simulink model "Hunt_crossley_MCMC"  (Simulink 8.9)
settings: Solver=ode3  StartTime=0.0  StopTime=25  FixedStep=0.001  RelTol=1e-3  EnableMultiTasking=on
undefined symbols (not defined in the file): sigbuilder_block
libraries: simulink x3, dspstat3 x1
settings Model: Creator=x  LastModifiedBy=x
settings DataIOCC: SignalLoggingSaveFormat=Dataset
settings OptimizationCC: ExpressionDepthLimit=2147483647
settings DebuggingCC: SolverPrmCheckMsg=warning  FcnCallInpInsideContextMsg=error
settings GRTTargetCC: CombineOutputUpdateFcns=on  GRTInterface=off

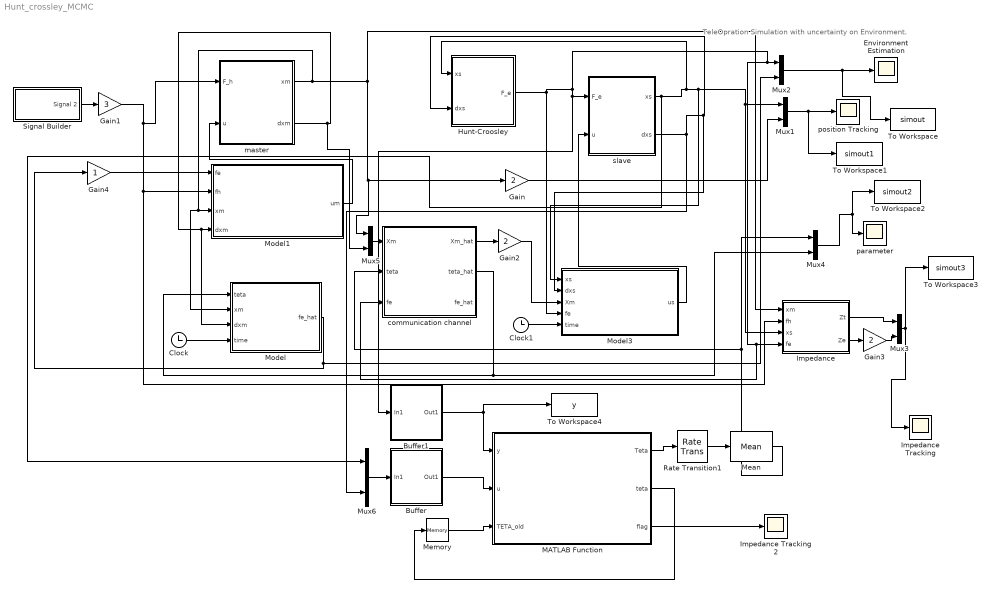
== system Hunt_crossley_MCMC ==
  note: TeleOpration Simulation with uncertainty on Environment.
  Buffer : Subsystem
  Buffer1 : Subsystem
  Clock : Clock
  Clock1 : Clock
  Environment Estimation : Scope
  Gain : Gain  Gain=2
  Gain1 : Gain  Gain=3
  Gain2 : Gain  Gain=2
  Gain3 : Gain  Gain=2
  Gain4 : Gain
  Hunt-Croosley : Subsystem
  Impedance : MATLAB Function  TreatAsAtomicUnit=on
  "Impedance Tracking " : Scope
  Impedance Tracking 2 : Scope
  MATLAB Function : MATLAB Function  TreatAsAtomicUnit=on
  Mean : dspstat3/Mean  run=off  reset_popup=None  InputProcessing=Columns as channels (frame based)  directionMode=Each row  dimension=1  roiEnable=off  roiType=Rectangles  roiPortion=Entire ROI  roiOutput=Individual statistics for each ROI  roiFlag=off  outputDataTypeStr=Inherit: Same as accumulator  outputLastDataTypeStr=Inherit: Same as accumulator  outputMin=[]  outputMax=[]  roundingMode=Floor  overflowMode=off
  Memory : Memory  X0=[1;1 ;1]*ones(1,2000)  InheritSampleTime=on
  Model : MATLAB Function  TreatAsAtomicUnit=on
  Model1 : MATLAB Function  TreatAsAtomicUnit=on
  Model3 : MATLAB Function  TreatAsAtomicUnit=on
  Mux{1..6} (6 alike) : Mux  Inputs=2
  Rate Transition1 : RateTransition  OutPortSampleTime=0.001
  Signal Builder : Subsystem  Tag=STV Subsys  LoadFcn=sigbuilder_block('load');  StartFcn=sigbuilder_block('start');  StopFcn=sigbuilder_block('stop');  ClipboardFcn=sigbuilder_block('clipboard');  mask(Sigbuilder block){tuvar=[0:10]}
      mask help: Simulink:masks:SigbuilderBlock_MD
      mask init:
      | if ~strcmp(get_param(bdroot(gcbh),'SimulationStatus'),'stopped') tuvar = sigbuilder_block('maskInit'); end
      settings: CopyFcn=sigbuilder_block('copy');  DeleteFcn=sigbuilder_block('delete');  ModelCloseFcn=sigbuilder_block('modelClose');  PreSaveFcn=sigbuilder_block('preSave');  PauseFcn=sigbuilder_block('pause');  ContinueFcn=sigbuilder_block('continue');  NameChangeFcn=sigbuilder_block('namechange');  OpenFcn=sigbuilder_block('open',[216 34.1379 544.345 383.586 ]);  CloseFcn=sigbuilder_block('close');
      mask Display: plot(0, 0, 100, 100,[2, 2, 32, 32, 2], [68, 8, 8, 68, 68],[32, 2], [38, 38], [32, 19, 2],[53, 60, 44], [32, 17, 17, 2],[16, 16, 31, 31]);txt = getActiveGroup(gcbh);text(2, 100, txt,'verticalAlignment', 'top');
  To Workspace : ToWorkspace  VariableName=simout  SampleTime=-1
  To Workspace1 : ToWorkspace  VariableName=simout1  SampleTime=-1
  To Workspace2 : ToWorkspace  VariableName=simout2  SampleTime=-1
  To Workspace3 : ToWorkspace  VariableName=simout3  SampleTime=-1
  To Workspace4 : ToWorkspace  VariableName=y  SampleTime=-1
  communication channel : Subsystem
  master : Subsystem
  parameter : Scope
  position Tracking : Scope
  slave : Subsystem
  wires:
  master/1(xm) -> Model/2(xm), Model1/3(xm), Mux5/1, Gain/1, Impedance/1(xm)
  Gain/1 -> Mux1/2
  Mux1/1 -> To Workspace1/1, position Tracking/1
  Impedance/1(Zt) -> Mux3/1
  Mux3/1 -> To Workspace3/1, "Impedance Tracking "/1
  communication channel/1(Xm_hat) -> Gain2/1
  Impedance/2(Ze) -> Gain3/1
  Signal Builder/1(Signal 2) -> Gain1/1
  Gain3/1 -> Mux3/2
  Model1/1(um) -> master/2(u)
  Model3/1(us) -> slave/2(u)
  master/2(dxm) -> Mux5/2, Model/3(dxm), Model1/4(dxm)
  Gain2/1 -> Model3/3(Xm)
  Clock/1 -> Model/4(time)
  communication channel/2(teta_hat) -> Mux4/2, Model/1(teta)
  Mean/1 -> Mux4/1, communication channel/2(teta)
  Mux5/1 -> communication channel/1(Xm)
  Clock1/1 -> Model3/5(time)
  Mux2/1 -> To Workspace/1, Environment Estimation/1
  Mux4/1 -> To Workspace2/1, parameter/1
  Gain1/1 -> master/1(F_h), Model1/2(fh), Impedance/2(fh)
  Model/1(fe_hat) -> Gain4/1, Mux2/2
  Gain4/1 -> Model1/1(fe)
  Mux6/1 -> Buffer/1(In1)
  MATLAB Function/2(teta) -> Memory/1
  Buffer/1(Out1) -> MATLAB Function/2(u)
  Buffer1/1(Out1) -> MATLAB Function/1(y), To Workspace4/1
  Rate Transition1/1 -> Mean/1
  Memory/1 -> MATLAB Function/3(TETA_old)
  MATLAB Function/1(Teta) -> Rate Transition1/1
  Hunt-Croosley/1(F_e) -> Buffer1/1(In1), slave/1(F_e), communication channel/3(fe), Impedance/4(fe), Mux2/1, Model3/4(fe)
  slave/1(xs) -> Mux6/1, Model3/1(xs), Impedance/3(xs), Mux1/1, Hunt-Croosley/1(xs)
  slave/2(dxs) -> Mux6/2, Model3/2(dxs), Hunt-Croosley/2(dxs)
  MATLAB Function/3(flag) -> Impedance Tracking 2/1

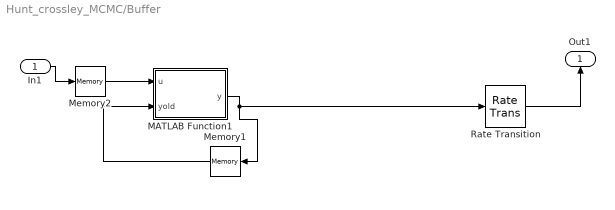
== system Hunt_crossley_MCMC/Buffer ==
  In1 : Inport
  MATLAB Function1 : MATLAB Function  TreatAsAtomicUnit=on
  Memory1 : Memory  X0=zeros(100,2)  LinearizeMemory=on
  Memory2 : Memory  X0=[0;0]  InheritSampleTime=on
  Rate Transition : RateTransition  X0=zeros(100,2)  OutPortSampleTime=0.1
  Out1 : Outport
  wires:
  Rate Transition/1 -> Out1/1
  Memory1/1 -> MATLAB Function1/2(yold)
  In1/1 -> Memory2/1
  MATLAB Function1/1(y) -> Memory1/1, Rate Transition/1
  Memory2/1 -> MATLAB Function1/1(u)

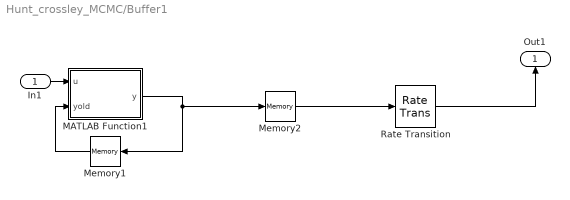
== system Hunt_crossley_MCMC/Buffer1 ==
  In1 : Inport
  MATLAB Function1 : MATLAB Function  TreatAsAtomicUnit=on
  Memory1 : Memory  X0=zeros(100,1)  LinearizeMemory=on
  Memory2 : Memory  X0=zeros(100,1)  LinearizeMemory=on
  Rate Transition : RateTransition  X0=zeros(100,1)  OutPortSampleTime=0.1
  Out1 : Outport
  wires:
  Memory1/1 -> MATLAB Function1/2(yold)
  In1/1 -> MATLAB Function1/1(u)
  Rate Transition/1 -> Out1/1
  MATLAB Function1/1(y) -> Memory2/1, Memory1/1
  Memory2/1 -> Rate Transition/1

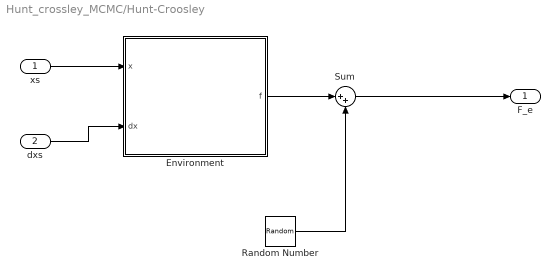
== system Hunt_crossley_MCMC/Hunt-Croosley ==
  xs : Inport
  dxs : Inport  Port=2
  Environment : MATLAB Function  TreatAsAtomicUnit=on
  Random Number : RandomNumber  Variance=0.1
  Sum : Sum  Inputs=|++
  F_e : Outport
  wires:
  xs/1 -> Environment/1(x)
  dxs/1 -> Environment/2(dx)
  Environment/1(f) -> Sum/1
  Sum/1 -> F_e/1
  Random Number/1 -> Sum/2

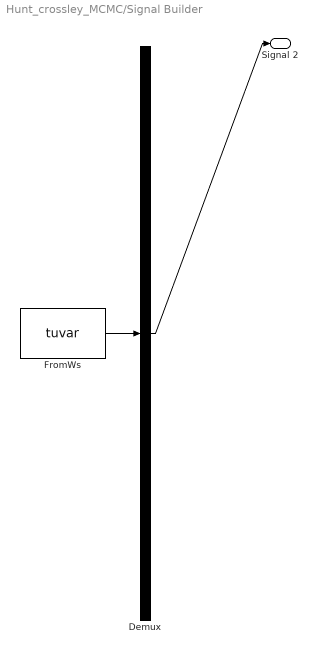
== system Hunt_crossley_MCMC/Signal Builder ==
  Demux : Demux  Tag=STV Demux  Outputs=1
  FromWs : FromWorkspace  Tag=STV FromWs  VariableName=tuvar  SampleTime=0  SigBuilderData=DataTag1  VnvData=DataTag2
      SigBuilderData=|
      | common.afterFinalStr = 'Extrapolate'
      | common.sampleTime = 0
      | dataSet.timeRange = [0 25]
      | dataSet.name = 'Group 1'
      | sbobj.Groups.Name = 'Group 1'
      | sbobj.Groups.Signals.Name = 'Signal 2'
      | sbobj.Groups.Signals.XData = [0 5.05 5.05 15.05 15.05 16.35 16.35 21.05 21.05 25]
      | sbobj.Groups.Signals.YData = [0.49 0.49 1.98 1.98 -0.82 -0.82 0.98 0.98 -0.24 -0.24]
      | sbobj.Groups.TimeRange = [0 25]
  Signal 2 : Outport  Tag=STV Outport
  wires:
  FromWs/1 -> Demux/1
  Demux/1 -> Signal 2/1

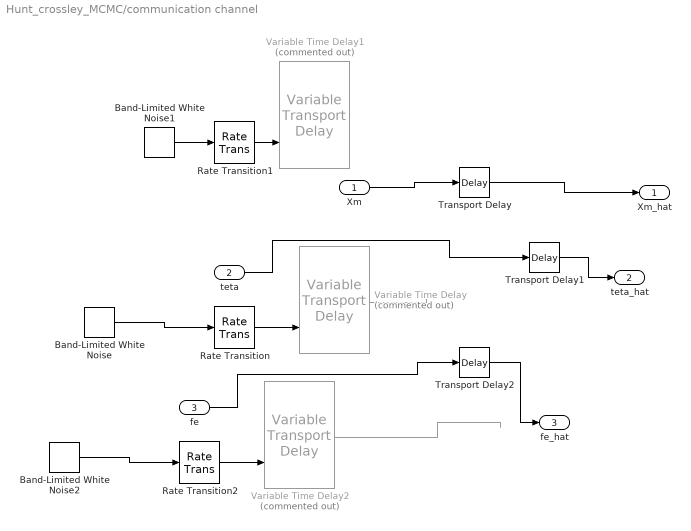
== system Hunt_crossley_MCMC/communication channel ==
  Xm : Inport
  teta : Inport  Port=2
  fe : Inport  Port=3
  Band-Limited White Noise : simulink/Sources/Band-Limited White Noise  Cov=[0.1]  Ts=0.2  seed=[23341]
  Band-Limited White Noise1 : simulink/Sources/Band-Limited White Noise  Cov=[0.1]  Ts=0.2  seed=[5368541]
  Band-Limited White Noise2 : simulink/Sources/Band-Limited White Noise  Cov=[0.1]  Ts=0.2  seed=[28931]
  Rate Transition : RateTransition
  Rate Transition1 : RateTransition
  Rate Transition2 : RateTransition
  Transport Delay : TransportDelay
  Transport Delay1 : TransportDelay
  Transport Delay2 : TransportDelay
  Variable Time Delay : VariableTransportDelay  Commented=on  MaximumDelay=4  TransDelayFeedthrough=on
  Variable Time Delay1 : VariableTransportDelay  Commented=on  MaximumDelay=4  TransDelayFeedthrough=on
  Variable Time Delay2 : VariableTransportDelay  Commented=on  MaximumDelay=4  TransDelayFeedthrough=on
  Xm_hat : Outport
  teta_hat : Outport  Port=2
  fe_hat : Outport  Port=3
  wires:
  Band-Limited White Noise/1 -> Rate Transition/1
  Rate Transition/1 -> Variable Time Delay/2
  Band-Limited White Noise1/1 -> Rate Transition1/1
  Rate Transition1/1 -> Variable Time Delay1/2
  Variable Time Delay/1 -> ?
  Band-Limited White Noise2/1 -> Rate Transition2/1
  Rate Transition2/1 -> Variable Time Delay2/2
  Variable Time Delay2/1 -> ?
  fe/1 -> Transport Delay2/1
  Xm/1 -> Transport Delay/1
  Transport Delay/1 -> Xm_hat/1
  Transport Delay1/1 -> teta_hat/1
  teta/1 -> Transport Delay1/1
  Transport Delay2/1 -> fe_hat/1

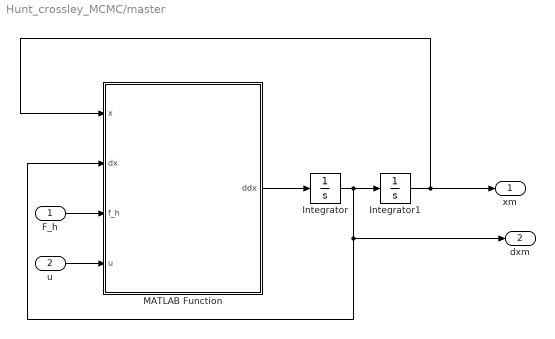
== system Hunt_crossley_MCMC/master ==
  F_h : Inport
  u : Inport  Port=2
  Integrator : Integrator
  Integrator1 : Integrator
  MATLAB Function : MATLAB Function  TreatAsAtomicUnit=on
  xm : Outport
  dxm : Outport  Port=2
  wires:
  F_h/1 -> MATLAB Function/3(f_h)
  u/1 -> MATLAB Function/4(u)
  MATLAB Function/1(ddx) -> Integrator/1
  Integrator/1 -> dxm/1, MATLAB Function/2(dx), Integrator1/1
  Integrator1/1 -> MATLAB Function/1(x), xm/1

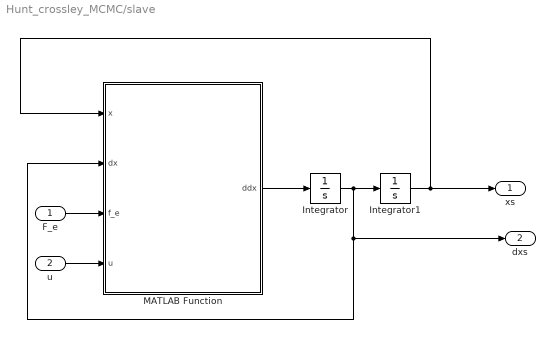
== system Hunt_crossley_MCMC/slave ==
  F_e : Inport
  u : Inport  Port=2
  Integrator : Integrator
  Integrator1 : Integrator
  MATLAB Function : MATLAB Function  TreatAsAtomicUnit=on
  xs : Outport
  dxs : Outport  Port=2
  wires:
  F_e/1 -> MATLAB Function/3(f_e)
  u/1 -> MATLAB Function/4(u)
  MATLAB Function/1(ddx) -> Integrator/1
  Integrator/1 -> dxs/1, MATLAB Function/2(dx), Integrator1/1
  Integrator1/1 -> xs/1, MATLAB Function/1(x)

== matlab function slave/MATLAB Function ==
  data: x input double; dx input double; f_e input double; u input double; ddx output double
function ddx = fcn(x,dx,f_e,u)
%parameter
ms=0.07; bs=0.05;ks=0.08; 
ms=1; bs=0.5;ks=0.8; 

ddx=ms^-1*(u-f_e-bs*dx-ks*x);

== matlab function master/MATLAB Function ==
  data: x input double; dx input double; f_h input double; u input double; ddx output double
function ddx = fcn(x,dx,f_h,u)
%parameter
jm=0.05; bm=0.03;km=0.1; l_eff=0.5;

ddx=jm^-1*(u+f_h*l_eff-bm*dx-km*x);

== matlab function Impedance ==
  data: xm input double; fh input double; xs input double; Zt output double; fe input double; Ze output double
function [Zt,Ze] = impedance(xm,fh,xs,fe)
%control parameter
if xm<1e-3 && xm>-1e-3
    Zt=0;
else 
    Zt=fh/xm;
end
if xs<1e-3
   Ze=0;
else
    Ze=fe/xs;
end

== matlab function Hunt-Croosley/Environment ==
  data: x input double; dx input double; f output double
function f= ENV( x,dx )
%   Parameter
K=4;B=2.3; n=1.7;

if x<0
    f=0;
else
    f=(x^n)*(K+B*dx);
end

end

== matlab function Model ==
  data: teta input double; fe_hat output double; xm input double; dxm input double; time input double
function fe_hat= ENV_Model( teta ,xm,dxm,time)
%   Parameter
kp=2;
if time==0.001
fe_hat=0;
else
if xm<0
   fe_hat=0;
else
    K=teta(1);B=teta(2); n=teta(3);
    fe_hat=(kp*xm)^n*(K+B*(kp*dxm));
end
end
end

== matlab function Model1 ==
  data: fe input double; um output double; fh input double; xm input double; dxm input double
function um= Master_Impedance_control( fe,fh,xm,dxm )
%   Parameter
jm=0.05; bm=0.03;km=0.1; l_eff=0.5;
% jmd=0.6; bmd=4;kmd=2;
% 
% um=(bm-jm/jmd*bmd)*dxm+(km-jm/jmd*kmd)*xm+(jm/jmd)*(fh-fe)-l_eff*fh;

jmd=0.6*20; bmd=4*2;kmd=2*2;

um=(bm-jm/jmd*bmd)*dxm+(km-jm/jmd*kmd)*xm+(jm/jmd)*(fh-fe)-l_eff*fh;

end

== matlab function Model3 ==
  data: xs input double; dxs input double; Xm input double; fe input double; us output double; time input double
function us= slave_Impedance_control( xs,dxs,Xm,fe,time )
%   Parameter
ms=1; bs=0.5;ks=0.8; 
jsd=50; bsd=150;ksd=100;
if time==0.001
    us=0;
else
xm=Xm(1);
dxm=Xm(2);
us=-(ms/jsd*bsd)*(dxs-dxm)-(ms/jsd*ksd)*(xs-xm)+(1-0*ms/jsd)*fe+bs*dxs+ks*xs;
end
end

== matlab function Buffer/MATLAB Function1 ==
  data: u input double; y output double; yold input double
function y = fcn(u,yold)
%#codegen

y = [yold(2:100,:);u'];

== matlab function Buffer1/MATLAB Function1 ==
  data: u input double; y output double; yold input double
function y = fcn(u,yold)
%#codegen

y = [yold(2:100);u];

== matlab function MATLAB Function ==
  data: Teta output double; y input double; u input double; TETA_old input double; teta output double; flag output double
function [Teta,teta,flag]  = online_enhanced_mcmc(y,u,TETA_old)
coder.extrinsic('ksdensity');
coder.extrinsic('unifrnd');
kde_y=zeros(1,100);
kde_x=zeros(1,100);
kde=zeros(2,100);
n=100;
lambda=0.95;
SampNum=2000;
nac=0;
count = 0;
ParNum = 3;
sigma2_RW = .000001;
sigma2_RW = .01;
sigma2 = 0.03;   
% preallcoation for speed
epsi=zeros(ParNum, 1);
ye1=0;
flag=0; %noninformative prior
inint_ths=10^22;
inint_ths=10^(-200000);
init_low=1.5;
init_high=4.5;
SampMin=1500;
AccMin=0.5;
npdf=1/sqrt(2*pi*sigma2^2);

ye1_candid = 0;

%%%%%%%%%%%%%%%%%%%%%%%%%%%% special cases (flag=2)%%%%%%%%%%%%%%%%%%%%%%%%%%%%%%%%%%%
% no environment
for i2 = 1:n
    if (u(i2,1)<0 && u(i2,2)<0 ) || (u(i2,1)<-0.001*sqrt(sigma2)*rand)
        count=count+1*0*(exp(-lambda*(n-i2)))+1;
    end
end
% start up
if min(y)==0 && max(y)==0 
    teta=TETA_old;
    flag=2;
    
elseif count>0.05*n
    teta=TETA_old*0;
    flag=2;
else
 u(:,1)=abs(u(:,1));
%%%%%%%%%%%%%%%%%%%%%%%%%%%% Normal cases (flag!=2)%%%%%%%%%%%%%%%%%%%%%%%%%%%%%%%%%%%
  %--------------------- Initializing -----------------------------------
dummy=0;
teta=[TETA_old(:,2:end), (mean(TETA_old(:,floor(SampNum/2):end)'))'];
for i2 = 1:n
    %ye1(i2) = u(i2,:) * teta(:,end) ;
    dumm=teta(1,end)+teta(2,end)*u(i2,2);
    if dumm <0
        dummy=-inf;
        break;
    end
    ye1 = teta(3,end)*log10(u(i2,1))+log10(dumm) ;
    dummy=log10(npdf*exp(-(exp(-lambda*(n-i2)))*(y(i2) - 10^ye1)^2/sigma2^2))+dummy;
    %dummy = log10(normpdf(y(i2) - ye1(i2), 0, sigma2)) + dummy;
end

if 10^dummy>inint_ths
    prob_teta = dummy;
    
%%%%%%%%%%%%%%%%%%%% informative prior (flag=1)%%%%%%%%%%%%%%%%%%%%%%%%%%
    
    sigma2_RW=0.003*sigma2_RW;
 for  k = 1:SampNum
      
        %-------------------- Introducing Candidate ---------------------------
%                          epsi(:,k) = teta(:,k) + normrnd(0,sqrt(sigma2_RW),[size(teta,1),1]);
                            epsi= teta(:,ceil(rand*ParNum))+sqrt(sigma2_RW)*randn([size(teta,1),1]); 
                            

        %-------------------- Evaluating Acceptance ---------------------------

        % Prior Knowledg
        if ( epsi(1)>4.5) ||( epsi(1)<3.5) || (epsi(2)> 3) ||(epsi(2)< 2) ||  ( epsi(3) > 2)||(epsi(3)< 1) 
            prob_epsi = -inf;
        else

            ye1_candid = 0;
            dummy = 0; % Computing Probability of Epsilon Parameter
            for i2 = 1:n
                % ---- Computing candidate probability accordance to noise distribution ----

%                 ye1_candid(i2) =  u(i2,:) * epsi(:);
                 dumm= epsi(1)+epsi(2)*u(i2,2);
                 if dumm<0
                     dummy=-inf;
                     break;
                 end
                ye1_candid = epsi(3)*log10(u(i2,1))+log10(dumm) ;
                

                %dummy = log10(normpdf(y(i2) - ye1_candid(i2), 0,sigma2)) + dummy;
                dummy=log10(npdf*exp(-(exp(-lambda*(n-i2)))*(y(i2) - 10^ye1_candid)^2/sigma2^2))+dummy;

            end

            prob_epsi = dummy;

        end
        alpha = min(1,10^(prob_epsi-prob_teta));
        z = rand(1,1);
        
            if (z < alpha)
                teta = [teta(:,2:end), epsi];
                prob_teta = prob_epsi;
                nac=nac+1;
            else
                teta = [teta(:,2:end), teta(:,end)];
            end
            
            if (k>SampMin && nac <k*AccMin)
                break;
            end
            if (k==floor(0.75*SampMin) && nac <0.5*k*AccMin)
                sigma2_RW=0.1*sigma2_RW;
            end
            if (k==0.5*SampMin && nac <0.5*k*AccMin)
                sigma2_RW=0.1*sigma2_RW;
            end
      
 end
   
   flag=1; 
end




%%%%%%%%%%%%%%%%%%%% non informative prior (flag=0)%%%%%%%%%%%%%%%%%%%%%%%%%%
if flag==0
dummy = -inf;
while (isinf(dummy))
% while (10^dummy<1e-10)
    teta(:,1) = unifrnd(init_low,init_high,[ParNum,1]);
    teta(2,1) = unifrnd(3.5,4.1);
    teta(2,1) = unifrnd(2,2.5);
    teta(3,1) = unifrnd(1,2);
    dummy = 0; % Computing Probability of Previous Sample Parameter
            
   % ye1 = 0; 
            
    for i2 = 1:n

%            ye1(i2) = u(i2,:) * teta(:,1);
            dumm = teta(1,1)+teta(2,1)*u(i2,2);
            if dumm<0
                dummy=-inf;
                break;
            end
           ye1 = teta(3,1)*log10(u(i2,1))+log10(dumm) ;
                    % -------- Computing first step of MCMC accordance to noise type ------
           %dummy = log10(normpdf(y(i2) - ye1(i2), 0, sigma2)) + dummy ;
           dummy=log10(npdf*exp(-(exp(-lambda*(n-i2)))*(y(i2) - 10^ye1)^2/sigma2^2))+dummy;

           if isinf(dummy)
                 break;
           end

    end

    prob_teta = dummy; 
%     count = count + 1
end

for  k = 1:(SampNum-1)
    
    prob_teta = dummy;
      
        %-------------------- Introducing Candidate ---------------------------
                     
               epsi = teta(:,k) +sqrt(sigma2_RW)*randn([size(teta,1),1]);
                      
        %-------------------- Evaluating Acceptance ---------------------------
          % Prior Knowledg
        if ( epsi(1)>4.5 ) ||( epsi(1)<3.5 ) || (epsi(2)> 3) ||(epsi(2)< 2) ||  ( epsi(3) > 2)||(epsi(3)< 1) 
            prob_epsi = -inf;
        else

            ye1_candid = 0;
            dummy = 0; % Computing Probability of Epsilon Parameter
            for i2 = 1:n
                % ---- Computing candidate probability accordance to noise distribution ----

%                 ye1_candid(i2) =  u(i2,:) * epsi(:);

                dumm = epsi(1)+epsi(2)*u(i2,2);
            if dumm<0
                dummy=-inf;
                break;
            end
                ye1_candid = epsi(3)*log10(u(i2,1))+log10(dumm) ;

                %dummy = log10(normpdf(y(i2) - ye1_candid(i2), 0,sigma2)) + dummy;
                dummy=log10(npdf*exp(-(exp(-lambda*(n-i2)))*(y(i2) - 10^ye1_candid)^2/sigma2^2))+dummy;

            end

            prob_epsi = dummy;

        end

        alpha = min(1,10^(prob_epsi-prob_teta));
        z = rand(1,1);
        
            if (z < alpha)
                teta(:,k+1) = epsi;
                prob_teta = prob_epsi;
                nac=nac+1;
            else
                teta(:,k+1) = teta(:,k);
            end
            
           % if (k>2*SampMin && nac<0.5*k*AccMin)
           %     break;
           % end
            if (k==floor(1.5*SampMin) && nac <0.5*k*AccMin)
                sigma2_RW=0.5*sigma2_RW;
            end
            if (k==2*SampMin && nac <0.8*k*AccMin)
                sigma2_RW=0.5*sigma2_RW;
            end
end
end
    
%nac=nac/k;
end


 [kde_x,kde_y]=ksdensity(teta(1,500:end));
 kde=[kde_x ;kde_y];
 %figure(1);
 plot(kde_y ,kde_x);
% [kde_x,kde_y]=ksdensity(teta(2,500:end));
%%figure(2);
%%plot(kde_y ,kde_x);
%[kde_x,kde_y]=ksdensity(teta(3,500:end));
%figure(3);
%plot(kde_y ,kde_x);
Teta=teta(:,500:end);
end
